simulink model "Pendulum_Simulink_CoreyO"  (R2020a)
settings: Solver=VariableStepAuto  StartTime=0.0  StopTime=30  MaxStep=.1  RelTol=1e-3
libraries: simulink x3
settings Model: DataTypeOverride=Double  MinMaxOverflowLogging=ForceOff  Creator=cjobr  LastModifiedBy=cjobr

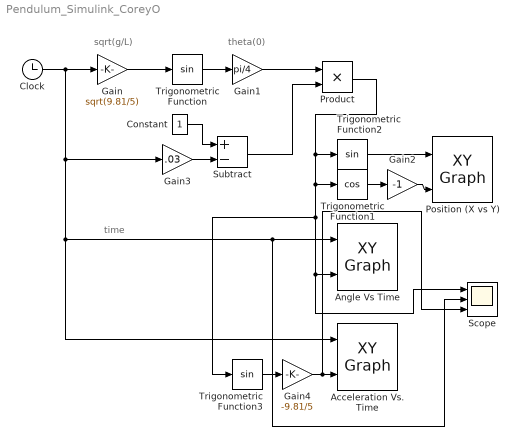
== system Pendulum_Simulink_CoreyO ==
  note: time
  note: theta(0)
  note: sqrt(g/L)
  Acceleration Vs. Time : simulink/Sinks/XY Graph  xmin=-1  xmax=35  ymin=-3  ymax=3  st=-1
  Angle Vs Time : simulink/Sinks/XY Graph  xmin=-1  xmax=35  ymin=-1  ymax=1  st=-1
  Clock : Clock
  Constant : Constant
  Gain : Gain  Gain=sqrt(9.81/5)
  Gain1 : Gain  Gain=pi/4
  Gain2 : Gain  Gain=-1
  Gain3 : Gain  Gain=.03
  Gain4 : Gain  Gain=-9.81/5
  Position (X vs Y) : simulink/Sinks/XY Graph  xmin=-1  xmax=1  ymin=-1  ymax=1  st=-1
  Product : Product
  Scope : Scope  NumInputPorts=3
  Subtract : Sum  Inputs=+-
  Trigonometric Function : Trigonometry
  Trigonometric Function1 : Trigonometry  Operator=cos
  Trigonometric Function2 : Trigonometry
  Trigonometric Function3 : Trigonometry
  wires:
  Clock/1 -> Gain3/1, Acceleration Vs. Time/1, Angle Vs Time/1, Scope/2, Gain/1
  Gain/1 -> Trigonometric Function/1
  Trigonometric Function/1 -> Gain1/1
  Trigonometric Function2/1 -> Position (X vs Y)/1
  Trigonometric Function1/1 -> Gain2/1
  Gain2/1 -> Position (X vs Y)/2
  Gain1/1 -> Product/1
  Gain3/1 -> Subtract/2
  Constant/1 -> Subtract/1
  Subtract/1 -> Product/2
  Product/1 -> Trigonometric Function3/1, Scope/1, Angle Vs Time/2, Trigonometric Function1/1, Trigonometric Function2/1
  Trigonometric Function3/1 -> Gain4/1
  Gain4/1 -> Scope/3, Acceleration Vs. Time/2
